simulink model "HVDCMMCInterconnection"  (R2024b)
settings: Solver=FixedStepDiscrete  StartTime=0.0  StopTime=11  RelTol=1e-3
PreLoadFcn:
  | GFLParameters_400Kv
  | HVDCMMCInterconnectionParam
StartFcn:
  | tic
StopFcn:
  | toc
values from neighbouring files (symbols this model uses):
  C_PM = 1.758e-3    (= 0.001758)    [HVDCMMCInterconnectionParam.m]
  Cfilter = 1/(Larm*wc2)    (= 4.78421193241e-05)    [HVDCMMCInterconnectionParam.m]
  Cg = 50e-9    (= 5e-08)    [HVDCMMCInterconnectionParam.m]
  Fc = Fnom*3.37    (= 168.5)    [HVDCMMCInterconnectionParam.m]
  Fnom = 50    [GFLParameters_400Kv.m]    (also in HVDCMMCInterconnectionParam.m)
  L_cable = 15e-3    (= 0.015)    [HVDCMMCInterconnectionParam.m]
  Larm = Larm_pu*(Zbase/(2*pi*Fnom))    (= 0.0529455974536)    [HVDCMMCInterconnectionParam.m]
  Limits_Qreg = [ 0.25, -0.25 ]    [HVDCMMCInterconnectionParam.m]
  Lxfo = 0.12    [HVDCMMCInterconnectionParam.m]
  Nb_PM = 36    [HVDCMMCInterconnectionParam.m]
  Pnom = 1000e6    (= 1000000000)    [HVDCMMCInterconnectionParam.m]
  Psc = Pnom*20    (= 20000000000)    [HVDCMMCInterconnectionParam.m]    (also in HVDCMMC_RunFaultAnalysis.m = gridSCLArray(k))
  R_cable = 0.5    [HVDCMMCInterconnectionParam.m]
  R_startup = 400    [HVDCMMCInterconnectionParam.m]
  Rarm = Rarm_pu*Zbase    (= 0.1663335)    [HVDCMMCInterconnectionParam.m]
  Rfilter = 1/(Cfilter*w)*30    (= 1996.002)    [HVDCMMCInterconnectionParam.m]
  Rg = 100    [HVDCMMCInterconnectionParam.m]
  Rxfo = 0.003    [HVDCMMCInterconnectionParam.m]
  Slope_Pref = 0.5    [HVDCMMCInterconnectionParam.m]
  Slope_Qref = 0.5    [HVDCMMCInterconnectionParam.m]
  Slope_Vdc_ref = Vnom_dc/5    (= 128000)    [HVDCMMCInterconnectionParam.m]
  Tbrk1_On = 0.1    [HVDCMMCInterconnectionParam.m]
  Tbrk2_On = 1.0    (= 1)    [HVDCMMCInterconnectionParam.m]
  Tdeblock = 1.5    [HVDCMMCInterconnectionParam.m]
  Tfault = 9999    [HVDCMMCInterconnectionParam.m]
  Ton_Converter2 = 4    [HVDCMMCInterconnectionParam.m]
  Ton_PQreg = 4    [HVDCMMCInterconnectionParam.m]
  Ton_VDCreg = 1.5    [HVDCMMCInterconnectionParam.m]
  Ts = Ts_Control    (= 4e-05)    [HVDCMMCInterconnectionParam.m]
  Ts_Power = 20e-6    (= 2e-05)    [HVDCMMCInterconnectionParam.m]
  Vnom_dc = 640e3    (= 640000)    [HVDCMMCInterconnectionParam.m]
  Vnom_prim = 400e3    (= 400000)    [HVDCMMCInterconnectionParam.m]
  Vnom_sec = 333e3    (= 333000)    [HVDCMMCInterconnectionParam.m]
undefined symbols (not defined in the file or in its folder): ConvCtrl, ConvPlt, DiscIntNeverNeededParam, Discrete, ee_sli_rtmsupport, Fault, gcbh, gridInverter, magnitude, Pcc, PlantSim, sps, sps_rtmsupport, spsPLL3phModel, TL, Trf
libraries: powerlib_extras x27, spsSeriesRLCBranchLib x27, simulink x14, eeGeneralControl x11, spsCurrentMeasurementLib x11, spsVoltageMeasurementLib x8, spsBreakerLib x7, eeTransforms x6, spsHalfBridgeMMCLib x6, spsSecondOrderFilterLib x4, spsabctodq0Lib x4, spsThreePhaseVIMeasurementLib x4
(part 2 of 6)

== system HVDCMMCInterconnection/Subsystem2 ==
  Current Measurement1 : spsCurrentMeasurementLib/Current Measurement  PhasorSimulation=off  OutputType=Complex  PSBequivalent=0
  Voltage Measurement : spsVoltageMeasurementLib/Voltage Measurement  PhasorSimulation=off  OutputType=Complex  PSBequivalent=0
  I1 : PMIOPort  Side=Left
  I2 : PMIOPort  Port=2  Side=Left
  O1 : PMIOPort  Port=3  Side=Right
  O2 : PMIOPort  Port=4  Side=Right
  tag scope: I_Bp=global, V12_Bp=global
  wires:
  Voltage Measurement/1 -> [V12_Bp]
  Current Measurement1/1 -> [I_Bp]
  connections:
  Voltage Measurement/LConn2 -- O2/RConn1 -- I2/RConn1
  Current Measurement1/LConn1 -- O1/RConn1
  Voltage Measurement/LConn1 -- Current Measurement1/RConn1 -- I1/RConn1

== system HVDCMMCInterconnection/Subsystem3 ==
  Current Measurement1 : spsCurrentMeasurementLib/Current Measurement  PhasorSimulation=off  OutputType=Complex  PSBequivalent=0
  Voltage Measurement : spsVoltageMeasurementLib/Voltage Measurement  PhasorSimulation=off  OutputType=Complex  PSBequivalent=0
  I1 : PMIOPort  Side=Left
  I2 : PMIOPort  Port=2  Side=Left
  O1 : PMIOPort  Port=3  Side=Right
  O2 : PMIOPort  Port=4  Side=Right
  tag scope: I_Bm=global, V12_Bm=global
  wires:
  Current Measurement1/1 -> [I_Bm]
  Voltage Measurement/1 -> [V12_Bm]
  connections:
  I1/RConn1 -- Current Measurement1/RConn1 -- Voltage Measurement/LConn1
  Current Measurement1/LConn1 -- O1/RConn1
  I2/RConn1 -- O2/RConn1 -- Voltage Measurement/LConn2

== system HVDCMMCInterconnection/Subsystem4 ==
  Current Measurement1 : spsCurrentMeasurementLib/Current Measurement  PhasorSimulation=off  OutputType=Complex  PSBequivalent=0
  Voltage Measurement : spsVoltageMeasurementLib/Voltage Measurement  PhasorSimulation=off  OutputType=Complex  PSBequivalent=0
  I1 : PMIOPort  Side=Left
  I2 : PMIOPort  Port=2  Side=Left
  O1 : PMIOPort  Port=3  Side=Right
  O2 : PMIOPort  Port=4  Side=Right
  tag scope: I_Cp=global, V12_Cp=global
  wires:
  Current Measurement1/1 -> [I_Cp]
  Voltage Measurement/1 -> [V12_Cp]
  connections:
  I1/RConn1 -- Current Measurement1/RConn1 -- Voltage Measurement/LConn1
  Current Measurement1/LConn1 -- O1/RConn1
  I2/RConn1 -- O2/RConn1 -- Voltage Measurement/LConn2

== system HVDCMMCInterconnection/Subsystem5 ==
  Current Measurement1 : spsCurrentMeasurementLib/Current Measurement  PhasorSimulation=off  OutputType=Complex  PSBequivalent=0
  Voltage Measurement : spsVoltageMeasurementLib/Voltage Measurement  PhasorSimulation=off  OutputType=Complex  PSBequivalent=0
  I1 : PMIOPort  Side=Left
  I2 : PMIOPort  Port=2  Side=Left
  O1 : PMIOPort  Port=3  Side=Right
  O2 : PMIOPort  Port=4  Side=Right
  tag scope: I_Cm=global, V12_Cm=global
  wires:
  Voltage Measurement/1 -> [V12_Cm]
  Current Measurement1/1 -> [I_Cm]
  connections:
  Voltage Measurement/LConn2 -- O2/RConn1 -- I2/RConn1
  Current Measurement1/LConn1 -- O1/RConn1
  Voltage Measurement/LConn1 -- Current Measurement1/RConn1 -- I1/RConn1

== system HVDCMMCInterconnection/param ==

== system HVDCMMCInterconnection/BusCalculations/Complex2Phasor ==
  complex : Inport
  Bus Creator1 : BusCreator  Inputs=3
  Bus Creator2 : BusCreator  Inputs=2
  Bus Creator3 : BusCreator  Inputs=2
  Bus Creator5 : BusCreator  Inputs=2
  Complex to Magnitude-Angle3 : ComplexToMagnitudeAngle
  Demux2 : Demux  Outputs=3
  Demux3 : Demux  Outputs=3
  Gain : Gain  Gain=180/pi
  Phasor : Outport
  wires:
  complex/1 -> Complex to Magnitude-Angle3/1
  Demux2/3 -> Bus Creator3/1  "mag"
  Complex to Magnitude-Angle3/1 -> Demux2/1
  Demux3/2 -> Bus Creator5/2  "phase"
  Demux2/1 -> Bus Creator2/1  "mag"
  Complex to Magnitude-Angle3/2 -> Gain/1
  Demux2/2 -> Bus Creator5/1  "mag"
  Demux3/1 -> Bus Creator2/2  "phase"
  Demux3/3 -> Bus Creator3/2  "phase"
  Bus Creator2/1 -> Bus Creator1/1  "a"
  Bus Creator5/1 -> Bus Creator1/2  "b"
  Bus Creator3/1 -> Bus Creator1/3  "c"
  Bus Creator1/1 -> Phasor/1  "Phasor"
  Gain/1 -> Demux3/1

== system HVDCMMCInterconnection/BusCalculations/Complex2Phasor1 ==
  complex : Inport
  Bus Creator1 : BusCreator  Inputs=3
  Bus Creator2 : BusCreator  Inputs=2
  Bus Creator3 : BusCreator  Inputs=2
  Bus Creator5 : BusCreator  Inputs=2
  Complex to Magnitude-Angle3 : ComplexToMagnitudeAngle
  Demux2 : Demux  Outputs=3
  Demux3 : Demux  Outputs=3
  Gain : Gain  Gain=180/pi
  Phasor : Outport
  wires:
  Bus Creator1/1 -> Phasor/1  "Phasor"
  Bus Creator3/1 -> Bus Creator1/3  "c"
  Bus Creator5/1 -> Bus Creator1/2  "b"
  Bus Creator2/1 -> Bus Creator1/1  "a"
  Demux3/3 -> Bus Creator3/2  "phase"
  Demux3/1 -> Bus Creator2/2  "phase"
  Demux2/2 -> Bus Creator5/1  "mag"
  Complex to Magnitude-Angle3/2 -> Gain/1
  Demux2/1 -> Bus Creator2/1  "mag"
  Demux3/2 -> Bus Creator5/2  "phase"
  Complex to Magnitude-Angle3/1 -> Demux2/1
  Demux2/3 -> Bus Creator3/1  "mag"
  complex/1 -> Complex to Magnitude-Angle3/1
  Gain/1 -> Demux3/1

== system HVDCMMCInterconnection/BusCalculations/Measurement Unit (Phasor Computation) ==
  Vabc(t) : Inport  PortDimensions=3
  Iabc(t) : Inport  Port=2  PortDimensions=3
  Demux : Demux  Outputs=3
      settings: DisplayOption=none
  Demux1 : Demux  Outputs=3
      settings: DisplayOption=none
  Discrete Fourier(A) : Subsystem  AncestorBlock=|  mask(Discrete Fourier){Freq=Freq, n=1, Par_Init=[0 0], Ts=Ts}
      | powerlib_extras/Discrete
      | Measurements/Discrete 
      | Fourier
      mask prompts: Freq "Fundamental frequency (Hz):"; n "Harmonic n (0=DC; 1=fundamental; 2=2nd harm;  ...):"; Par_Init "Initial input: [ Mag  Phase(degrees) ]"; Ts "Sample time:"
      mask help:
      | This block computes the fundamental value of the input signal over a running window of one cycle of the specified fundamental frequency. First and second outputs return respectively the magnitude and phase (degrees) of the fundamental.
      | For the first cycle of simulation, the ouputs are held constant to the value specified by the parameter "Initial input".
      mask init:
      | k=2-(n==0);
      | SamplesPerCycle=1/Freq/Ts;
      | RoundSamplesPerCycle=round(SamplesPerCycle);
      | Delay=RoundSamplesPerCycle*Ts - Ts/2;
      | Correction=SamplesPerCycle/RoundSamplesPerCycle - 1;
      | Real_Init=Par_Init(1)*cos(pi/180*Par_Init(2));
      | Imag_Init=Par_Init(1)*sin(pi/180*Par_Init(2));
  "Discrete Fourier(A) " : Subsystem  AncestorBlock=|  mask(Discrete Fourier){Freq=Freq, n=1, Par_Init=[0 0], Ts=Ts}
      | powerlib_extras/Discrete
      | Measurements/Discrete 
      | Fourier
      mask prompts: Freq "Fundamental frequency (Hz):"; n "Harmonic n (0=DC; 1=fundamental; 2=2nd harm;  ...):"; Par_Init "Initial input: [ Mag  Phase(degrees) ]"; Ts "Sample time:"
      mask help:
      | This block computes the fundamental value of the input signal over a running window of one cycle of the specified fundamental frequency. First and second outputs return respectively the magnitude and phase (degrees) of the fundamental.
      | For the first cycle of simulation, the ouputs are held constant to the value specified by the parameter "Initial input".
      mask init: same as HVDCMMCInterconnection/BusCalculations/Measurement Unit (Phasor Computation)/Discrete Fourier(A)
  Discrete Fourier(B) : Subsystem  AncestorBlock=|  mask(Discrete Fourier){Freq=Freq, n=1, Par_Init=[0 -120], Ts=Ts}
      | powerlib_extras/Discrete
      | Measurements/Discrete 
      | Fourier
      mask prompts: Freq "Fundamental frequency (Hz):"; n "Harmonic n (0=DC; 1=fundamental; 2=2nd harm;  ...):"; Par_Init "Initial input: [ Mag  Phase(degrees) ]"; Ts "Sample time:"
      mask help:
      | This block computes the fundamental value of the input signal over a running window of one cycle of the specified fundamental frequency. First and second outputs return respectively the magnitude and phase (degrees) of the fundamental.
      | For the first cycle of simulation, the ouputs are held constant to the value specified by the parameter "Initial input".
      mask init: same as HVDCMMCInterconnection/BusCalculations/Measurement Unit (Phasor Computation)/Discrete Fourier(A)
  "Discrete Fourier(B) " : Subsystem  AncestorBlock=|  mask(Discrete Fourier){Freq=Freq, n=1, Par_Init=[0 -120], Ts=Ts}
      | powerlib_extras/Discrete
      | Measurements/Discrete 
      | Fourier
      mask prompts: Freq "Fundamental frequency (Hz):"; n "Harmonic n (0=DC; 1=fundamental; 2=2nd harm;  ...):"; Par_Init "Initial input: [ Mag  Phase(degrees) ]"; Ts "Sample time:"
      mask help:
      | This block computes the fundamental value of the input signal over a running window of one cycle of the specified fundamental frequency. First and second outputs return respectively the magnitude and phase (degrees) of the fundamental.
      | For the first cycle of simulation, the ouputs are held constant to the value specified by the parameter "Initial input".
      mask init: same as HVDCMMCInterconnection/BusCalculations/Measurement Unit (Phasor Computation)/Discrete Fourier(A)
  Discrete Fourier(C) : Subsystem  AncestorBlock=|  mask(Discrete Fourier){Freq=Freq, n=1, Par_Init=[0 120], Ts=Ts}
      | powerlib_extras/Discrete
      | Measurements/Discrete 
      | Fourier
      mask prompts: Freq "Fundamental frequency (Hz):"; n "Harmonic n (0=DC; 1=fundamental; 2=2nd harm;  ...):"; Par_Init "Initial input: [ Mag  Phase(degrees) ]"; Ts "Sample time:"
      mask help:
      | This block computes the fundamental value of the input signal over a running window of one cycle of the specified fundamental frequency. First and second outputs return respectively the magnitude and phase (degrees) of the fundamental.
      | For the first cycle of simulation, the ouputs are held constant to the value specified by the parameter "Initial input".
      mask init: same as HVDCMMCInterconnection/BusCalculations/Measurement Unit (Phasor Computation)/Discrete Fourier(A)
  "Discrete Fourier(C) " : Subsystem  AncestorBlock=|  mask(Discrete Fourier){Freq=Freq, n=1, Par_Init=[0 120], Ts=Ts}
      | powerlib_extras/Discrete
      | Measurements/Discrete 
      | Fourier
      mask prompts: Freq "Fundamental frequency (Hz):"; n "Harmonic n (0=DC; 1=fundamental; 2=2nd harm;  ...):"; Par_Init "Initial input: [ Mag  Phase(degrees) ]"; Ts "Sample time:"
      mask help:
      | This block computes the fundamental value of the input signal over a running window of one cycle of the specified fundamental frequency. First and second outputs return respectively the magnitude and phase (degrees) of the fundamental.
      | For the first cycle of simulation, the ouputs are held constant to the value specified by the parameter "Initial input".
      mask init: same as HVDCMMCInterconnection/BusCalculations/Measurement Unit (Phasor Computation)/Discrete Fourier(A)
  Mux : Mux  Inputs=3
  Mux1 : Mux  Inputs=3
  Vabc_Fund : Outport
  " Iabc_Fund" : Outport  Port=2
  wires:
  "Discrete Fourier(C) "/1(Fund) -> Mux1/3
  "Discrete Fourier(B) "/1(Fund) -> Mux1/2
  "Discrete Fourier(A) "/1(Fund) -> Mux1/1
  Mux1/1 -> " Iabc_Fund"/1
  Iabc(t)/1 -> Demux1/1
  Demux1/3 -> "Discrete Fourier(C) "/1(In)
  Demux1/2 -> "Discrete Fourier(B) "/1(In)
  Demux1/1 -> "Discrete Fourier(A) "/1(In)
  Mux/1 -> Vabc_Fund/1
  Discrete Fourier(C)/1(Fund) -> Mux/3
  Discrete Fourier(B)/1(Fund) -> Mux/2
  Discrete Fourier(A)/1(Fund) -> Mux/1
  Demux/3 -> Discrete Fourier(C)/1(In)
  Demux/2 -> Discrete Fourier(B)/1(In)
  Vabc(t)/1 -> Demux/1
  Demux/1 -> Discrete Fourier(A)/1(In)

== system HVDCMMCInterconnection/BusCalculations/SymmetricalComponentsCalc ==
  abc : Inport
  Bus Creator{,1..4,7..8} (7 alike) : BusCreator  Inputs=3
  Bus Creator5 : BusCreator  Inputs=2
  Bus Creator6 : BusCreator  Inputs=2
  Bus Creator9 : BusCreator  Inputs=2
  Complex to Magnitude-Angle1 : ComplexToMagnitudeAngle
  Complex to Magnitude-Angle2 : ComplexToMagnitudeAngle
  Complex to Magnitude-Angle3 : ComplexToMagnitudeAngle
  Demux{,1..5} (6 alike) : Demux  Outputs=3
  Gain : Gain  Gain=[exp(1i*4*pi/3) 0 0; 0 exp(1i*2*pi/3) 0; 0 0 1]  Multiplication=Matrix(K*u)
  Gain1 : Gain  Gain=[exp(1i*2*pi/3) 0 0; 0 exp(1i*4*pi/3) 0; 0 0 1]  Multiplication=Matrix(K*u)
  Gain2 : Gain  Gain=180/pi
  Gain3 : Gain  Gain=180/pi
  Gain4 : Gain  Gain=180/pi
  Symmetrical-Components Transform1 : eeTransforms/Symmetrical-Components Transform  PowerInvariant=off
  ABC+-0 : Outport
  wires:
  Demux/2 -> Bus Creator3/2  "neg"
  Complex to Magnitude-Angle3/2 -> Gain2/1
  Demux/1 -> Bus Creator3/1  "pos"
  Symmetrical-Components Transform1/1 -> Complex to Magnitude-Angle3/1, Gain/1, Gain1/1
  Demux/3 -> Bus Creator3/3  "zero"
  Bus Creator3/1 -> Bus Creator5/1  "mag"
  Complex to Magnitude-Angle3/1 -> Demux/1
  Bus Creator4/1 -> Bus Creator5/2  "phase"
  abc/1 -> Symmetrical-Components Transform1/1
  Bus Creator5/1 -> Bus Creator/1  "A"
  Bus Creator6/1 -> Bus Creator/2  "B"
  Bus Creator2/1 -> Bus Creator6/2  "phase"
  Complex to Magnitude-Angle1/1 -> Demux2/1
  Bus Creator1/1 -> Bus Creator6/1  "mag"
  Complex to Magnitude-Angle1/2 -> Gain3/1
  Gain/1 -> Complex to Magnitude-Angle1/1
  Complex to Magnitude-Angle2/2 -> Gain4/1
  Bus Creator7/1 -> Bus Creator9/1  "mag"
  Complex to Magnitude-Angle2/1 -> Demux4/1
  Bus Creator8/1 -> Bus Creator9/2  "phase"
  Bus Creator9/1 -> Bus Creator/3  "C"
  Gain1/1 -> Complex to Magnitude-Angle2/1
  Bus Creator/1 -> ABC+-0/1
  Demux1/1 -> Bus Creator4/1  "pos"
  Demux1/3 -> Bus Creator4/3  "zero"
  Demux1/2 -> Bus Creator4/2  "neg"
  Demux2/2 -> Bus Creator1/2  "neg"
  Demux2/3 -> Bus Creator1/3  "zero"
  Demux2/1 -> Bus Creator1/1  "pos"
  Demux3/2 -> Bus Creator2/2  "neg"
  Demux3/3 -> Bus Creator2/3  "zero"
  Demux3/1 -> Bus Creator2/1  "pos"
  Demux4/2 -> Bus Creator7/2  "neg"
  Demux4/3 -> Bus Creator7/3  "zero"
  Demux4/1 -> Bus Creator7/1  "pos"
  Demux5/2 -> Bus Creator8/2  "neg"
  Demux5/3 -> Bus Creator8/3  "zero"
  Demux5/1 -> Bus Creator8/1  "pos"
  Gain2/1 -> Demux1/1
  Gain3/1 -> Demux3/1
  Gain4/1 -> Demux5/1

== system HVDCMMCInterconnection/BusCalculations/SymmetricalComponentsCalc1 ==
  abc : Inport
  Bus Creator{,1..4,7..8} (7 alike) : BusCreator  Inputs=3
  Bus Creator5 : BusCreator  Inputs=2
  Bus Creator6 : BusCreator  Inputs=2
  Bus Creator9 : BusCreator  Inputs=2
  Complex to Magnitude-Angle1 : ComplexToMagnitudeAngle
  Complex to Magnitude-Angle2 : ComplexToMagnitudeAngle
  Complex to Magnitude-Angle3 : ComplexToMagnitudeAngle
  Demux{,1..5} (6 alike) : Demux  Outputs=3
  Gain : Gain  Gain=[exp(1i*4*pi/3) 0 0; 0 exp(1i*2*pi/3) 0; 0 0 1]  Multiplication=Matrix(K*u)
  Gain1 : Gain  Gain=[exp(1i*2*pi/3) 0 0; 0 exp(1i*4*pi/3) 0; 0 0 1]  Multiplication=Matrix(K*u)
  Gain2 : Gain  Gain=180/pi
  Gain3 : Gain  Gain=180/pi
  Gain4 : Gain  Gain=180/pi
  Symmetrical-Components Transform1 : eeTransforms/Symmetrical-Components Transform  PowerInvariant=off
  ABC+-0 : Outport
  wires:
  Gain4/1 -> Demux5/1
  Gain3/1 -> Demux3/1
  Gain2/1 -> Demux1/1
  Demux5/1 -> Bus Creator8/1  "pos"
  Demux5/3 -> Bus Creator8/3  "zero"
  Demux5/2 -> Bus Creator8/2  "neg"
  Demux4/1 -> Bus Creator7/1  "pos"
  Demux4/3 -> Bus Creator7/3  "zero"
  Demux4/2 -> Bus Creator7/2  "neg"
  Demux3/1 -> Bus Creator2/1  "pos"
  Demux3/3 -> Bus Creator2/3  "zero"
  Demux3/2 -> Bus Creator2/2  "neg"
  Demux2/1 -> Bus Creator1/1  "pos"
  Demux2/3 -> Bus Creator1/3  "zero"
  Demux2/2 -> Bus Creator1/2  "neg"
  Demux1/2 -> Bus Creator4/2  "neg"
  Demux1/3 -> Bus Creator4/3  "zero"
  Demux1/1 -> Bus Creator4/1  "pos"
  Bus Creator/1 -> ABC+-0/1
  Gain1/1 -> Complex to Magnitude-Angle2/1
  Bus Creator9/1 -> Bus Creator/3  "C"
  Bus Creator8/1 -> Bus Creator9/2  "phase"
  Complex to Magnitude-Angle2/1 -> Demux4/1
  Bus Creator7/1 -> Bus Creator9/1  "mag"
  Complex to Magnitude-Angle2/2 -> Gain4/1
  Gain/1 -> Complex to Magnitude-Angle1/1
  Complex to Magnitude-Angle1/2 -> Gain3/1
  Bus Creator1/1 -> Bus Creator6/1  "mag"
  Complex to Magnitude-Angle1/1 -> Demux2/1
  Bus Creator2/1 -> Bus Creator6/2  "phase"
  Bus Creator6/1 -> Bus Creator/2  "B"
  Bus Creator5/1 -> Bus Creator/1  "A"
  abc/1 -> Symmetrical-Components Transform1/1
  Bus Creator4/1 -> Bus Creator5/2  "phase"
  Complex to Magnitude-Angle3/1 -> Demux/1
  Bus Creator3/1 -> Bus Creator5/1  "mag"
  Demux/3 -> Bus Creator3/3  "zero"
  Symmetrical-Components Transform1/1 -> Gain1/1, Gain/1, Complex to Magnitude-Angle3/1
  Demux/1 -> Bus Creator3/1  "pos"
  Complex to Magnitude-Angle3/2 -> Gain2/1
  Demux/2 -> Bus Creator3/2  "neg"

== system HVDCMMCInterconnection/BusCalculations1/Complex2Phasor ==
  complex : Inport
  Bus Creator1 : BusCreator  Inputs=3
  Bus Creator2 : BusCreator  Inputs=2
  Bus Creator3 : BusCreator  Inputs=2
  Bus Creator5 : BusCreator  Inputs=2
  Complex to Magnitude-Angle3 : ComplexToMagnitudeAngle
  Demux2 : Demux  Outputs=3
  Demux3 : Demux  Outputs=3
  Gain : Gain  Gain=180/pi
  Phasor : Outport
  wires:
  Gain/1 -> Demux3/1
  Bus Creator1/1 -> Phasor/1  "Phasor"
  Bus Creator3/1 -> Bus Creator1/3  "c"
  Bus Creator5/1 -> Bus Creator1/2  "b"
  Bus Creator2/1 -> Bus Creator1/1  "a"
  Demux3/3 -> Bus Creator3/2  "phase"
  Demux3/1 -> Bus Creator2/2  "phase"
  Demux2/2 -> Bus Creator5/1  "mag"
  Complex to Magnitude-Angle3/2 -> Gain/1
  Demux2/1 -> Bus Creator2/1  "mag"
  Demux3/2 -> Bus Creator5/2  "phase"
  Complex to Magnitude-Angle3/1 -> Demux2/1
  Demux2/3 -> Bus Creator3/1  "mag"
  complex/1 -> Complex to Magnitude-Angle3/1

== system HVDCMMCInterconnection/BusCalculations1/Complex2Phasor1 ==
  complex : Inport
  Bus Creator1 : BusCreator  Inputs=3
  Bus Creator2 : BusCreator  Inputs=2
  Bus Creator3 : BusCreator  Inputs=2
  Bus Creator5 : BusCreator  Inputs=2
  Complex to Magnitude-Angle3 : ComplexToMagnitudeAngle
  Demux2 : Demux  Outputs=3
  Demux3 : Demux  Outputs=3
  Gain : Gain  Gain=180/pi
  Phasor : Outport
  wires:
  Gain/1 -> Demux3/1
  complex/1 -> Complex to Magnitude-Angle3/1
  Demux2/3 -> Bus Creator3/1  "mag"
  Complex to Magnitude-Angle3/1 -> Demux2/1
  Demux3/2 -> Bus Creator5/2  "phase"
  Demux2/1 -> Bus Creator2/1  "mag"
  Complex to Magnitude-Angle3/2 -> Gain/1
  Demux2/2 -> Bus Creator5/1  "mag"
  Demux3/1 -> Bus Creator2/2  "phase"
  Demux3/3 -> Bus Creator3/2  "phase"
  Bus Creator2/1 -> Bus Creator1/1  "a"
  Bus Creator5/1 -> Bus Creator1/2  "b"
  Bus Creator3/1 -> Bus Creator1/3  "c"
  Bus Creator1/1 -> Phasor/1  "Phasor"

== system HVDCMMCInterconnection/BusCalculations1/Measurement Unit (Phasor Computation) ==
  Vabc(t) : Inport  PortDimensions=3
  Iabc(t) : Inport  Port=2  PortDimensions=3
  Demux : Demux  Outputs=3
      settings: DisplayOption=none
  Demux1 : Demux  Outputs=3
      settings: DisplayOption=none
  Discrete Fourier(A) : Subsystem  AncestorBlock=|  mask(Discrete Fourier){Freq=Freq, n=1, Par_Init=[0 0], Ts=Ts}
      | powerlib_extras/Discrete
      | Measurements/Discrete 
      | Fourier
      mask prompts: Freq "Fundamental frequency (Hz):"; n "Harmonic n (0=DC; 1=fundamental; 2=2nd harm;  ...):"; Par_Init "Initial input: [ Mag  Phase(degrees) ]"; Ts "Sample time:"
      mask help:
      | This block computes the fundamental value of the input signal over a running window of one cycle of the specified fundamental frequency. First and second outputs return respectively the magnitude and phase (degrees) of the fundamental.
      | For the first cycle of simulation, the ouputs are held constant to the value specified by the parameter "Initial input".
      mask init: same as HVDCMMCInterconnection/BusCalculations/Measurement Unit (Phasor Computation)/Discrete Fourier(A)
  "Discrete Fourier(A) " : Subsystem  AncestorBlock=|  mask(Discrete Fourier){Freq=Freq, n=1, Par_Init=[0 0], Ts=Ts}
      | powerlib_extras/Discrete
      | Measurements/Discrete 
      | Fourier
      mask prompts: Freq "Fundamental frequency (Hz):"; n "Harmonic n (0=DC; 1=fundamental; 2=2nd harm;  ...):"; Par_Init "Initial input: [ Mag  Phase(degrees) ]"; Ts "Sample time:"
      mask help:
      | This block computes the fundamental value of the input signal over a running window of one cycle of the specified fundamental frequency. First and second outputs return respectively the magnitude and phase (degrees) of the fundamental.
      | For the first cycle of simulation, the ouputs are held constant to the value specified by the parameter "Initial input".
      mask init: same as HVDCMMCInterconnection/BusCalculations/Measurement Unit (Phasor Computation)/Discrete Fourier(A)
  Discrete Fourier(B) : Subsystem  AncestorBlock=|  mask(Discrete Fourier){Freq=Freq, n=1, Par_Init=[0 -120], Ts=Ts}
      | powerlib_extras/Discrete
      | Measurements/Discrete 
      | Fourier
      mask prompts: Freq "Fundamental frequency (Hz):"; n "Harmonic n (0=DC; 1=fundamental; 2=2nd harm;  ...):"; Par_Init "Initial input: [ Mag  Phase(degrees) ]"; Ts "Sample time:"
      mask help:
      | This block computes the fundamental value of the input signal over a running window of one cycle of the specified fundamental frequency. First and second outputs return respectively the magnitude and phase (degrees) of the fundamental.
      | For the first cycle of simulation, the ouputs are held constant to the value specified by the parameter "Initial input".
      mask init: same as HVDCMMCInterconnection/BusCalculations/Measurement Unit (Phasor Computation)/Discrete Fourier(A)
  "Discrete Fourier(B) " : Subsystem  AncestorBlock=|  mask(Discrete Fourier){Freq=Freq, n=1, Par_Init=[0 -120], Ts=Ts}
      | powerlib_extras/Discrete
      | Measurements/Discrete 
      | Fourier
      mask prompts: Freq "Fundamental frequency (Hz):"; n "Harmonic n (0=DC; 1=fundamental; 2=2nd harm;  ...):"; Par_Init "Initial input: [ Mag  Phase(degrees) ]"; Ts "Sample time:"
      mask help:
      | This block computes the fundamental value of the input signal over a running window of one cycle of the specified fundamental frequency. First and second outputs return respectively the magnitude and phase (degrees) of the fundamental.
      | For the first cycle of simulation, the ouputs are held constant to the value specified by the parameter "Initial input".
      mask init: same as HVDCMMCInterconnection/BusCalculations/Measurement Unit (Phasor Computation)/Discrete Fourier(A)
  Discrete Fourier(C) : Subsystem  AncestorBlock=|  mask(Discrete Fourier){Freq=Freq, n=1, Par_Init=[0 120], Ts=Ts}
      | powerlib_extras/Discrete
      | Measurements/Discrete 
      | Fourier
      mask prompts: Freq "Fundamental frequency (Hz):"; n "Harmonic n (0=DC; 1=fundamental; 2=2nd harm;  ...):"; Par_Init "Initial input: [ Mag  Phase(degrees) ]"; Ts "Sample time:"
      mask help:
      | This block computes the fundamental value of the input signal over a running window of one cycle of the specified fundamental frequency. First and second outputs return respectively the magnitude and phase (degrees) of the fundamental.
      | For the first cycle of simulation, the ouputs are held constant to the value specified by the parameter "Initial input".
      mask init: same as HVDCMMCInterconnection/BusCalculations/Measurement Unit (Phasor Computation)/Discrete Fourier(A)
  "Discrete Fourier(C) " : Subsystem  AncestorBlock=|  mask(Discrete Fourier){Freq=Freq, n=1, Par_Init=[0 120], Ts=Ts}
      | powerlib_extras/Discrete
      | Measurements/Discrete 
      | Fourier
      mask prompts: Freq "Fundamental frequency (Hz):"; n "Harmonic n (0=DC; 1=fundamental; 2=2nd harm;  ...):"; Par_Init "Initial input: [ Mag  Phase(degrees) ]"; Ts "Sample time:"
      mask help:
      | This block computes the fundamental value of the input signal over a running window of one cycle of the specified fundamental frequency. First and second outputs return respectively the magnitude and phase (degrees) of the fundamental.
      | For the first cycle of simulation, the ouputs are held constant to the value specified by the parameter "Initial input".
      mask init: same as HVDCMMCInterconnection/BusCalculations/Measurement Unit (Phasor Computation)/Discrete Fourier(A)
  Mux : Mux  Inputs=3
  Mux1 : Mux  Inputs=3
  Vabc_Fund : Outport
  " Iabc_Fund" : Outport  Port=2
  wires:
  Demux/1 -> Discrete Fourier(A)/1(In)
  Vabc(t)/1 -> Demux/1
  Demux/2 -> Discrete Fourier(B)/1(In)
  Demux/3 -> Discrete Fourier(C)/1(In)
  Discrete Fourier(A)/1(Fund) -> Mux/1
  Discrete Fourier(B)/1(Fund) -> Mux/2
  Discrete Fourier(C)/1(Fund) -> Mux/3
  Mux/1 -> Vabc_Fund/1
  Demux1/1 -> "Discrete Fourier(A) "/1(In)
  Demux1/2 -> "Discrete Fourier(B) "/1(In)
  Demux1/3 -> "Discrete Fourier(C) "/1(In)
  Iabc(t)/1 -> Demux1/1
  Mux1/1 -> " Iabc_Fund"/1
  "Discrete Fourier(A) "/1(Fund) -> Mux1/1
  "Discrete Fourier(B) "/1(Fund) -> Mux1/2
  "Discrete Fourier(C) "/1(Fund) -> Mux1/3

== system HVDCMMCInterconnection/BusCalculations1/SymmetricalComponentsCalc ==
  abc : Inport
  Bus Creator{,1..4,7..8} (7 alike) : BusCreator  Inputs=3
  Bus Creator5 : BusCreator  Inputs=2
  Bus Creator6 : BusCreator  Inputs=2
  Bus Creator9 : BusCreator  Inputs=2
  Complex to Magnitude-Angle1 : ComplexToMagnitudeAngle
  Complex to Magnitude-Angle2 : ComplexToMagnitudeAngle
  Complex to Magnitude-Angle3 : ComplexToMagnitudeAngle
  Demux{,1..5} (6 alike) : Demux  Outputs=3
  Gain : Gain  Gain=[exp(1i*4*pi/3) 0 0; 0 exp(1i*2*pi/3) 0; 0 0 1]  Multiplication=Matrix(K*u)
  Gain1 : Gain  Gain=[exp(1i*2*pi/3) 0 0; 0 exp(1i*4*pi/3) 0; 0 0 1]  Multiplication=Matrix(K*u)
  Gain2 : Gain  Gain=180/pi
  Gain3 : Gain  Gain=180/pi
  Gain4 : Gain  Gain=180/pi
  Symmetrical-Components Transform1 : eeTransforms/Symmetrical-Components Transform  PowerInvariant=off
  ABC+-0 : Outport
  wires:
  Gain4/1 -> Demux5/1
  Gain3/1 -> Demux3/1
  Gain2/1 -> Demux1/1
  Demux5/1 -> Bus Creator8/1  "pos"
  Demux5/3 -> Bus Creator8/3  "zero"
  Demux5/2 -> Bus Creator8/2  "neg"
  Demux4/1 -> Bus Creator7/1  "pos"
  Demux4/3 -> Bus Creator7/3  "zero"
  Demux4/2 -> Bus Creator7/2  "neg"
  Demux3/1 -> Bus Creator2/1  "pos"
  Demux3/3 -> Bus Creator2/3  "zero"
  Demux3/2 -> Bus Creator2/2  "neg"
  Demux2/1 -> Bus Creator1/1  "pos"
  Demux2/3 -> Bus Creator1/3  "zero"
  Demux2/2 -> Bus Creator1/2  "neg"
  Demux1/2 -> Bus Creator4/2  "neg"
  Demux1/3 -> Bus Creator4/3  "zero"
  Demux1/1 -> Bus Creator4/1  "pos"
  Bus Creator/1 -> ABC+-0/1
  Gain1/1 -> Complex to Magnitude-Angle2/1
  Bus Creator9/1 -> Bus Creator/3  "C"
  Bus Creator8/1 -> Bus Creator9/2  "phase"
  Complex to Magnitude-Angle2/1 -> Demux4/1
  Bus Creator7/1 -> Bus Creator9/1  "mag"
  Complex to Magnitude-Angle2/2 -> Gain4/1
  Gain/1 -> Complex to Magnitude-Angle1/1
  Complex to Magnitude-Angle1/2 -> Gain3/1
  Bus Creator1/1 -> Bus Creator6/1  "mag"
  Complex to Magnitude-Angle1/1 -> Demux2/1
  Bus Creator2/1 -> Bus Creator6/2  "phase"
  Bus Creator6/1 -> Bus Creator/2  "B"
  Bus Creator5/1 -> Bus Creator/1  "A"
  abc/1 -> Symmetrical-Components Transform1/1
  Bus Creator4/1 -> Bus Creator5/2  "phase"
  Complex to Magnitude-Angle3/1 -> Demux/1
  Bus Creator3/1 -> Bus Creator5/1  "mag"
  Demux/3 -> Bus Creator3/3  "zero"
  Symmetrical-Components Transform1/1 -> Gain1/1, Gain/1, Complex to Magnitude-Angle3/1
  Demux/1 -> Bus Creator3/1  "pos"
  Complex to Magnitude-Angle3/2 -> Gain2/1
  Demux/2 -> Bus Creator3/2  "neg"

== system HVDCMMCInterconnection/BusCalculations1/SymmetricalComponentsCalc1 ==
  abc : Inport
  Bus Creator{,1..4,7..8} (7 alike) : BusCreator  Inputs=3
  Bus Creator5 : BusCreator  Inputs=2
  Bus Creator6 : BusCreator  Inputs=2
  Bus Creator9 : BusCreator  Inputs=2
  Complex to Magnitude-Angle1 : ComplexToMagnitudeAngle
  Complex to Magnitude-Angle2 : ComplexToMagnitudeAngle
  Complex to Magnitude-Angle3 : ComplexToMagnitudeAngle
  Demux{,1..5} (6 alike) : Demux  Outputs=3
  Gain : Gain  Gain=[exp(1i*4*pi/3) 0 0; 0 exp(1i*2*pi/3) 0; 0 0 1]  Multiplication=Matrix(K*u)
  Gain1 : Gain  Gain=[exp(1i*2*pi/3) 0 0; 0 exp(1i*4*pi/3) 0; 0 0 1]  Multiplication=Matrix(K*u)
  Gain2 : Gain  Gain=180/pi
  Gain3 : Gain  Gain=180/pi
  Gain4 : Gain  Gain=180/pi
  Symmetrical-Components Transform1 : eeTransforms/Symmetrical-Components Transform  PowerInvariant=off
  ABC+-0 : Outport
  wires:
  Demux/2 -> Bus Creator3/2  "neg"
  Complex to Magnitude-Angle3/2 -> Gain2/1
  Demux/1 -> Bus Creator3/1  "pos"
  Symmetrical-Components Transform1/1 -> Complex to Magnitude-Angle3/1, Gain/1, Gain1/1
  Demux/3 -> Bus Creator3/3  "zero"
  Bus Creator3/1 -> Bus Creator5/1  "mag"
  Complex to Magnitude-Angle3/1 -> Demux/1
  Bus Creator4/1 -> Bus Creator5/2  "phase"
  abc/1 -> Symmetrical-Components Transform1/1
  Bus Creator5/1 -> Bus Creator/1  "A"
  Bus Creator6/1 -> Bus Creator/2  "B"
  Bus Creator2/1 -> Bus Creator6/2  "phase"
  Complex to Magnitude-Angle1/1 -> Demux2/1
  Bus Creator1/1 -> Bus Creator6/1  "mag"
  Complex to Magnitude-Angle1/2 -> Gain3/1
  Gain/1 -> Complex to Magnitude-Angle1/1
  Complex to Magnitude-Angle2/2 -> Gain4/1
  Bus Creator7/1 -> Bus Creator9/1  "mag"
  Complex to Magnitude-Angle2/1 -> Demux4/1
  Bus Creator8/1 -> Bus Creator9/2  "phase"
  Bus Creator9/1 -> Bus Creator/3  "C"
  Gain1/1 -> Complex to Magnitude-Angle2/1
  Bus Creator/1 -> ABC+-0/1
  Demux1/1 -> Bus Creator4/1  "pos"
  Demux1/3 -> Bus Creator4/3  "zero"
  Demux1/2 -> Bus Creator4/2  "neg"
  Demux2/2 -> Bus Creator1/2  "neg"
  Demux2/3 -> Bus Creator1/3  "zero"
  Demux2/1 -> Bus Creator1/1  "pos"
  Demux3/2 -> Bus Creator2/2  "neg"
  Demux3/3 -> Bus Creator2/3  "zero"
  Demux3/1 -> Bus Creator2/1  "pos"
  Demux4/2 -> Bus Creator7/2  "neg"
  Demux4/3 -> Bus Creator7/3  "zero"
  Demux4/1 -> Bus Creator7/1  "pos"
  Demux5/2 -> Bus Creator8/2  "neg"
  Demux5/3 -> Bus Creator8/3  "zero"
  Demux5/1 -> Bus Creator8/1  "pos"
  Gain2/1 -> Demux1/1
  Gain3/1 -> Demux3/1
  Gain4/1 -> Demux5/1

== system HVDCMMCInterconnection/Controllers/Controllers ==
  PrefPU : Inport
  QrefPU : Inport  Port=2
  Vdc : Inport  Port=3
  Vsec : Inport  Port=4
  Isec : Inport  Port=5
  VPcc : Inport  Port=6
  Grid-Following Converter Control : Subsystem  VariantControl=GFMGFLSelect == 0
  Grid-Forming Converter Control : Subsystem  VariantControl=GFMGFLSelect == 1  mask(Grid-Forming Controller){power=gridInverter.apparentPower, gridLineVoltage=gridInverter.lineRMSVoltage, powerFreq=gridInverter.frequency, dcBusVoltage=gridInverter.DCVoltage, measSampleTime=gridInverter.measurementSampleTime, powerControl=Virtual Synchronous Machine, activePowerSampleTime=gridInverter.droopControl.sampleTime, droopSlope=gridInverter.droopControl.freqSlopeMp, droopT1=gridInverter.droopControl.T1, droopT2=gridInverter.droopControl.T2, droopTC=gridInverter.droopControl.lpfTimeConst, vsmPmeasFilterTC=gridInverter.vsm.PmeasTimeConst, vsmFreqDroop=gridInverter.vsm.freqDroop, vsmInertiaTC=gridInverter.vsm.inertiaConstant, vsmDampingConst=gridInverter.vsm.dampingCoefficent, dampingPowerMaxLimit=gridInverter.vsm.maxDampingPower, dampingPowerMinLimit=gridInverter.vsm.minDampingPower, freqMeasTimeConst=gridInverter.freqMeasTimeConst, freqOption=Constant Frequency Reference, voltreference=gridInverter.Qcontrol.voltageReference, QVoltFilterTC=gridInverter.Qcontrol.QmeasTimeConst, QVoltDroop=gridInverter.Qcontrol.voltageDroop, lowVoltageSupportGain=gridInverter.Qcontrol.lowVoltageSupportGain, currentLimit=Virtual Impedance, maxSatCurrentLimit=gridInverter.currentLimit.maxSaturationCurrent, maxVICurrentLimit=gridInverter.currentLimit.viCurrentLimit, ctLimitVirtualImp=gridInverter.currentLimit.virImpResistanceCoeff, ctLimitXbyR=gridInverter.currentLimit.virImpXbyR, ctLimitDelayTime=gridInverter.currentLimit.maxSaturationDelay, currentSatTime=gridInverter.currentLimit.satCurrentRunTime, currentVITimeConst=gridInverter.currentLimit.viFilterTimeConst, modeTransferTime=10*gridInverter.controller.CurrentControlSampleTime, voltControlTs=gridInverter.controller.VoltageControlSampleTime, vdPGain=gridInverter.controller.voltControllerKp, VdIGain=gridInverter.controller.voltControllerKi, VdMaxCt=gridInverter.controller.voltageMaxId, VdMinCt=gridInverter.controller.voltageMinId, VqPGain=gridInverter.controller.voltControllerKp, VqIGain=gridInverter.controller.voltControllerKi, VqMaxCt=gridInverter.controller.voltageMaxIq, VqMinCt=gridInverter.controller.voltageMinIq, vdvqLPFTimeConst=gridInverter.controller.voltMeasTimeConst, currentControlTs=gridInverter.controller.CurrentControlSampleTime, filterInductance=gridInverter.L, IdPGain=gridInverter.controller.ctControllerKp, IdIGain=gridInverter.controller.ctControllerKi, IqPGain=gridInverter.controller.ctControllerKp, IqIGain=gridInverter.controller.ctControllerKi}
      mask prompts: power "Grid-forming converter power (VA)"; gridLineVoltage "Grid line voltage (V)"; powerFreq "Grid frequency (Hz)"; dcBusVoltage "DC bus voltage (V)"; measSampleTime "Measurement sample time (s)"; powerControl "Active Power Control"; activePowerSampleTime "Power controller sample time (s)"; droopSlope "Power droop slope (pu, Hz/W)"; droopT1 "Lead-Lag numerator time constant (s)"; droopT2 "Lead-Lag denominator time constant (s)"; droopTC "Filter cut-off time constant (s)"; vsmPmeasFilterTC "Power measurement filter time constant (s)"; vsmFreqDroop "Frequency droop (pu,  W/Hz)"; vsmInertiaTC "Inertia constant M (pu)"; vsmDampingConst "Damping constant (pu/Hz)"; dampingPowerMaxLimit "Damping power maximum limit (pu)"; dampingPowerMinLimit "Damping power minimum limit (pu)"; freqMeasTimeConst "Frequency measurement time constant (s)"; freqOption "Damping power frequency option"; voltreference "Voltage reference value (pu)"; QVoltFilterTC "Power measurement filter time constant (s)"; QVoltDroop "Voltage droop (pu, V/VAr)"; lowVoltageSupportGain "Low voltage support gain (pu, A/V)"; currentLimit "Current limiting method"; maxSatCurrentLimit "Maximum current saturation (pu)"; maxVICurrentLimit "Maximum virtual impedance current (pu)"; ctLimitVirtualImp "Virtual impedance coefficient (pu.Ohm/pu.A)"; ctLimitXbyR "Virtual X/R ratio"; ctLimitDelayTime "Maximum current delay time (s)"; currentSatTime "Current limiting run time (s)"; currentVITimeConst "Filter time constant (s)"; modeTransferTime "Mode transfer time (s)"; voltControlTs "Voltage controller sample time (s)"; vdPGain "Vd proportional gain"; VdIGain "Vd integral gain"; VdMaxCt "Vd maximum current limit (A)"; VdMinCt "Vd minimum current limit (A)"; VqPGain "Vq proportional gain"; VqIGain "Vq integral gain"; VqMaxCt "Vq maximum current limit (A)"; VqMinCt "Vq minimum current limit (A)"; vdvqLPFTimeConst "Voltage measurement filter time constant (s)"; currentControlTs "Current controller sample time (s)"; filterInductance "Filter inductance (H)"; IdPGain "Id proportional gain"; IdIGain "Id integral gain"; IqPGain "Iq proportional gain"; IqIGain "Iq integral gain"
      mask help: This block implements the grid forming controller with fault ride through capability. Input to the controller are active and reactive power reference in per unit and the sensed three-phase phase current in amphere and phase voltage in volts.
      mask init:
      | powerChoice = get_param(gcb,'powerControl');
      | currentChoice = get_param(gcb,'currentLimit');
      | 
      | powerloc = [gcb, '/Power Control/ActivePowerControl']; 
      | currentloc = [gcb, '/Current Limiting/CurrentLimitingMethod'];
      | freqLoc = [gcb,'/Power Control/ActivePowerControl/vsmControl/Damping Frequency'];
      | 
      | switch powerChoice
      |     case 'Virtual Synchronous Machine'
      |         set_param(powerloc, 'LabelModeActiveChoice', 'vsm');
      |         dampingFreqChoice = get_param(gcb,'freqOption');
      |         if strcmp(dampingFreqChoice,'Grid Frequency Measurement')
      |             set_param(freqLoc, 'LabelModeActiveChoice', 'freqMeas');
      |         else
      |             set_param(freqLoc, 'LabelModeActiveChoice', 'constFreq');
      |         end
      |     case 'Droop Control'
      |          set_param(powerloc, 'LabelModeActiveChoice', 'droop');
      |    otherwise
      |         disp('Choose proper active power control method')
      | end
      | switch currentChoice
      |     case 'Virtual Impedance'
      |           set_param(currentloc, 'LabelModeActiveChoice', 'virimp');
      |     case 'Current Limiting'
      |          set_param(currentloc, 'LabelModeActiveChoice', 'ctSat');
      |     case 'Virtual Impedance and Current Limiting'
      |             set_param(currentloc, 'LabelModeActiveChoice', 'both');
      |     otherwise
      |         disp('Choose proper current limiting method')
      | end
      mask Help: This block implements the grid forming controller with fault ride through capability. Input to the controller are active and reactive power reference in per unit and the sensed three-phase phase current in amphere and phase voltage in volts.
      mask TypeOptions powerControl: Virtual Synchronous Machine | Droop Control
      mask Callback powerControl:
      | h = Simulink.Mask.get(gcb);
      | slectedActivePowerControl=get_param(gcb,'powerControl');
      | %slectedActivePowerControl = h.Parameters(find(string({h.Parameters.Name}) == 'powerControl')).Value;
      | switch slectedActivePowerControl
      |     case 'Virtual Synchronous Machine'
      |         h.Parameters(find(string({h.Parameters.Name}) == 'droopSlope')).Visible = 'off';
      |         h.Parameters(find(string({h.Parameters.Name}) == 'droopTC')).Visible = 'off';
      |         h.Parameters(find(string({h.Parameters.Name}) == 'droopT1')).Visible = 'off';
      |         h.Parameters(find(string({h.Parameters.Name}) == 'droopT2')).Visible = 'off';
      |         h.Parameters(find(string({h.Parameters.Name}) == 'vsmPmeasFilterTC')).Visible = 'on';
      |         h.Parameters(find(string({h.Parameters.Name}) == 'vsmFreqDroop')).Visible = 'on';
      |         h.Parameters(find(string({h.Parameters.Name}) == 'vsmInertiaTC')).Visible = 'on';
      |         h.Parameters(find(string({h.Parameters.Name}) == 'vsmDampingConst')).Visible = 'on';
      |         h.Parameters(find(string({h.Parameters.Name}) == 'dampingPowerMaxLimit')).Visible = 'on';
      |         h.Parameters(find(string({h.Parameters.Name}) == 'dampingPowerMinLimit')).Visible = 'on';
      |         h.Parameters(find(string({h.Parameters.Name}) == 'freqOption')).Visible = 'on';
      |         h.Parameters(find(string({h.Parameters.Name}) == 'freqMeasTimeConst')).Visible = 'on';
      |     case 'Droop Control'
      |         h.Parameters(find(string({h.Parameters.Name}) == 'droopSlope')).Visible = 'on';
      |         h.Parameters(find(string({h.Parameters.Name}) == 'droopTC')).Visible = 'on';
      |         h.Parameters(find(string({h.Parameters.Name}) == 'droopT1')).Visible = 'on';
      |         h.Parameters(find(string({h.Parameters.Name}) == 'droopT2')).Visible = 'on';
      |         h.Parameters(find(string({h.Parameters.Name}) == 'vsmPmeasFilterTC')).Visible = 'off';
      |         h.Parameters(find(string({h.Parameters.Name}) == 'vsmFreqDroop')).Visible = 'off';
      |         h.Parameters(find(string({h.Parameters.Name}) == 'vsmInertiaTC')).Visible = 'off';
      |         h.Parameters(find(string({h.Parameters.Name}) == 'vsmDampingConst')).Visible = 'off';
      |         h.Parameters(find(string({h.Parameters.Name}) == 'dampingPowerMaxLimit')).Visible = 'off';
      |         h.Parameters(find(string({h.Parameters.Name}) == 'dampingPowerMinLimit')).Visible = 'off';
      |         h.Parameters(find(string({h.Parameters.Name}) == 'freqOption')).Visible = 'off';
      |         h.Parameters(find(string({h.Parameters.Name}) == 'freqMeasTimeConst')).Visible = 'on';
      | 
      |     otherwise
      |         disp('Choose proper active power control method')
      | end
      mask TypeOptions freqOption: Grid Frequency Measurement | Constant Frequency Reference
      mask TypeOptions currentLimit: Virtual Impedance | Current Limiting | Virtual Impedance and Current Limiting
      mask Callback currentLimit:
      | h = Simulink.Mask.get(gcb);
      | currentLimitControl=get_param(gcb,'currentLimit');
      | %slectedActivePowerControl = h.Parameters(find(string({h.Parameters.Name}) == 'powerControl')).Value;
      | switch currentLimitControl
      |     case 'Virtual Impedance'
      |         h.Parameters(find(string({h.Parameters.Name}) == 'maxVICurrentLimit')).Visible = 'on';
      |         h.Parameters(find(string({h.Parameters.Name}) == 'ctLimitVirtualImp')).Visible = 'on';
      |         h.Parameters(find(string({h.Parameters.Name}) == 'ctLimitXbyR')).Visible = 'on';
      |         h.Parameters(find(string({h.Parameters.Name}) == 'maxSatCurrentLimit')).Visible = 'off';
      |         h.Parameters(find(string({h.Parameters.Name}) == 'ctLimitDelayTime')).Visible = 'off';
      |         h.Parameters(find(string({h.Parameters.Name}) == 'currentSatTime')).Visible = 'off';
      |         h.Parameters(find(string({h.Parameters.Name}) == 'currentVITimeConst')).Visible = 'on';
      |         h.Parameters(find(string({h.Parameters.Name}) == 'modeTransferTime')).Visible = 'off';
      | 
      | 
      |     case 'Current Limiting'
      |         h.Parameters(find(string({h.Parameters.Name}) == 'maxVICurrentLimit')).Visible = 'off';
      |         h.Parameters(find(string({h.Parameters.Name}) == 'ctLimitVirtualImp')).Visible = 'off';
      |         h.Parameters(find(string({h.Parameters.Name}) == 'ctLimitXbyR')).Visible = 'off';
      |         h.Parameters(find(string({h.Parameters.Name}) == 'maxSatCurrentLimit')).Visible = 'on';
      |         h.Parameters(find(string({h.Parameters.Name}) == 'ctLimitDelayTime')).Visible = 'on';
      |         h.Parameters(find(string({h.Parameters.Name}) == 'currentSatTime')).Visible = 'off';
      |         h.Parameters(find(string({h.Parameters.Name}) == 'currentVITimeConst')).Visible = 'off';
      |         h.Parameters(find(string({h.Parameters.Name}) == 'modeTransferTime')).Visible = 'off';
      | 
      |     case 'Virtual Impedance and Current Limiting'
      |         h.Parameters(find(string({h.Parameters.Name}) == 'maxVICurrentLimit')).Visible = 'on';
      |         h.Parameters(find(string({h.Parameters.Name}) == 'ctLimitVirtualImp')).Visible = 'on';
      |         h.Parameters(find(string({h.Parameters.Name}) == 'ctLimitXbyR')).Visible = 'on';
      |         h.Parameters(find(string({h.Parameters.Name}) == 'maxSatCurrentLimit')).Visible = 'on';
      |         h.Parameters(find(string({h.Parameters.Name}) == 'ctLimitDelayTime')).Visible = 'off';
      |         h.Parameters(find(string({h.Parameters.Name}) == 'currentSatTime')).Visible = 'on';
      |         h.Parameters(find(string({h.Parameters.Name}) == 'currentVITimeConst')).Visible = 'on';
      |         h.Parameters(find(string({h.Parameters.Name}) == 'modeTransferTime')).Visible = 'on';
      | 
      |     otherwise
      |         disp('Choose proper current limiting method')
      | end
      mask DialogControl ParameterGroupVar Prompt: Grid-Forming Controller Parameters
      mask DialogControl GFMGroup Prompt: Grid-Forming Converter Specifications
      mask DialogControl Pcontrolgrp Prompt: Active Power Controller Parameters
      mask DialogControl QcontrolGrp Prompt: Reactive Power Controller Parameters
      mask DialogControl faultRideThroughGrp Prompt: Fault Ride-Through Parameters
      mask DialogControl voltControlgrp Prompt: Voltage Controller Parameters
      mask DialogControl Container15currentContGrp Prompt: Current Controller Parameters
      mask Display: image('$imagefile'); % Use "Edit Image" on toolstrip to change.
  Uref : Outport
  Pmeas : Outport  Port=2
  Qmeas : Outport  Port=3
  fmeas : Outport  Port=4
